simulink model "SecRwLtStHdrstUpwdDnwdTrgtPosSelc"  (R2018b)
settings: Solver=FixedStepDiscrete  StartTime=0.0  StopTime=10.0  FixedStep=0.01  RelTol=1e-3
undefined symbols (not defined in the file or in its folder): KeSMSw4SAcsMd21SecRwLtStHdrstUpwdDnwdPos_Val, KeSMSw4SAcsMd21SecRwLtStHdrstUpwdDnwdPosMax_Val, KeSMSw4SAcsMd21SecRwLtStHdrstUpwdDnwdPosMin_Val, KeSMSw4SAcsMd22SecRwLtStHdrstUpwdDnwdPos_Val, KeSMSw4SAcsMd22SecRwLtStHdrstUpwdDnwdPosMax_Val, KeSMSw4SAcsMd22SecRwLtStHdrstUpwdDnwdPosMin_Val, KeSMSw4SAcsMd25SecRwLtStHdrstUpwdDnwdPos_Val, KeSMSw4SAcsMd25SecRwLtStHdrstUpwdDnwdPosMax_Val, KeSMSw4SAcsMd25SecRwLtStHdrstUpwdDnwdPosMin_Val, KeSMSw4SAcsMd26SecRwLtStHdrstUpwdDnwdPos_Val, KeSMSw4SAcsMd26SecRwLtStHdrstUpwdDnwdPosMax_Val, KeSMSw4SAcsMd26SecRwLtStHdrstUpwdDnwdPosMin_Val, KeSMSw4sLyingMDSecRwLtStHdrstUpwdDnwdPos_160_Val, KeSMSw4sLyingMDSecRwLtStHdrstUpwdDnwdPos_165_Val, KeSMSw4sLyingMDSecRwLtStHdrstUpwdDnwdPos_170_Val, KeSMSw4sLyingMDSecRwLtStHdrstUpwdDnwdPos_175_Val, KeSMSw4sLyingMDSecRwLtStHdrstUpwdDnwdPos_180_Val, KeSMSw4sLyingMDSecRwLtStHdrstUpwdDnwdPos_Below160_Val, KeSMSw4sLyingMDSecRwLtStHdrstUpwdDnwdPos_Over180_Val, KeSMSw4sLyingMDSecRwLtStHdrstUpwdDnwdPosMax_160_Val, KeSMSw4sLyingMDSecRwLtStHdrstUpwdDnwdPosMax_165_Val, KeSMSw4sLyingMDSecRwLtStHdrstUpwdDnwdPosMax_170_Val, KeSMSw4sLyingMDSecRwLtStHdrstUpwdDnwdPosMax_175_Val, KeSMSw4sLyingMDSecRwLtStHdrstUpwdDnwdPosMax_180_Val, KeSMSw4sLyingMDSecRwLtStHdrstUpwdDnwdPosMax_Below160_Val, KeSMSw4sLyingMDSecRwLtStHdrstUpwdDnwdPosMax_Over180_Val, KeSMSw4sLyingMDSecRwLtStHdrstUpwdDnwdPosMin_160_Val, KeSMSw4sLyingMDSecRwLtStHdrstUpwdDnwdPosMin_165_Val, KeSMSw4sLyingMDSecRwLtStHdrstUpwdDnwdPosMin_170_Val, KeSMSw4sLyingMDSecRwLtStHdrstUpwdDnwdPosMin_175_Val, KeSMSw4sLyingMDSecRwLtStHdrstUpwdDnwdPosMin_180_Val, KeSMSw4sLyingMDSecRwLtStHdrstUpwdDnwdPosMin_Below160_Val, KeSMSw4sLyingMDSecRwLtStHdrstUpwdDnwdPosMin_Over180_Val, KeSMSw4sRecoveryMDSecRwLtStHdrstUpwdDnwdPos_160_Val, KeSMSw4sRecoveryMDSecRwLtStHdrstUpwdDnwdPos_165_Val, KeSMSw4sRecoveryMDSecRwLtStHdrstUpwdDnwdPos_170_Val, KeSMSw4sRecoveryMDSecRwLtStHdrstUpwdDnwdPos_175_Val, KeSMSw4sRecoveryMDSecRwLtStHdrstUpwdDnwdPos_180_Val, KeSMSw4sRecoveryMDSecRwLtStHdrstUpwdDnwdPos_Below160_Val, KeSMSw4sRecoveryMDSecRwLtStHdrstUpwdDnwdPos_Over180_Val, KeSMSw4sRecoveryMDSecRwLtStHdrstUpwdDnwdPosMax_160_Val, KeSMSw4sRecoveryMDSecRwLtStHdrstUpwdDnwdPosMax_165_Val, KeSMSw4sRecoveryMDSecRwLtStHdrstUpwdDnwdPosMax_170_Val, KeSMSw4sRecoveryMDSecRwLtStHdrstUpwdDnwdPosMax_175_Val, KeSMSw4sRecoveryMDSecRwLtStHdrstUpwdDnwdPosMax_180_Val, KeSMSw4sRecoveryMDSecRwLtStHdrstUpwdDnwdPosMax_Below160_Val, KeSMSw4sRecoveryMDSecRwLtStHdrstUpwdDnwdPosMax_Over180_Val, KeSMSw4sRecoveryMDSecRwLtStHdrstUpwdDnwdPosMin_160_Val, KeSMSw4sRecoveryMDSecRwLtStHdrstUpwdDnwdPosMin_165_Val, KeSMSw4sRecoveryMDSecRwLtStHdrstUpwdDnwdPosMin_170_Val, KeSMSw4sRecoveryMDSecRwLtStHdrstUpwdDnwdPosMin_175_Val, KeSMSw4sRecoveryMDSecRwLtStHdrstUpwdDnwdPosMin_180_Val, KeSMSw4sRecoveryMDSecRwLtStHdrstUpwdDnwdPosMin_Below160_Val, KeSMSw4sRecoveryMDSecRwLtStHdrstUpwdDnwdPosMin_Over180_Val, KeSMSw4sVIPMDSecRwLtStHdrstUpwdDnwdPos_160_Val, KeSMSw4sVIPMDSecRwLtStHdrstUpwdDnwdPos_165_Val, KeSMSw4sVIPMDSecRwLtStHdrstUpwdDnwdPos_170_Val, KeSMSw4sVIPMDSecRwLtStHdrstUpwdDnwdPos_175_Val, KeSMSw4sVIPMDSecRwLtStHdrstUpwdDnwdPos_180_Val, KeSMSw4sVIPMDSecRwLtStHdrstUpwdDnwdPos_Below160_Val ... (+15)
libraries: TrgtPosSelcLib x7
settings Model: ModifiedHistory=2023.8.1 V2.0.0 CR401790 增加模式21-26  Creator=sn2xws  LastModifiedBy=sn2xws
settings DataIOCC: SaveFormat=StructureWithTime
settings OptimizationCC: DefaultParameterBehavior=Inlined  EnhancedBackFolding=on  PassReuseOutputArgsAs=Individual arguments  ZeroExternalMemoryAtStartup=off  ZeroInternalMemoryAtStartup=off  OptimizeBlockOrder=speed  DifferentSizesBufferReuse=on  OptimizationCustomize=off
settings DebuggingCC: ParameterTunabilityLossMsg=error
settings ModelReferenceCC: ModelReferenceNumInstancesAllowed=Single
settings SFSimCC: MATLABDynamicMemAlloc=off
settings RTWCC: SystemTargetFile=autosar.tlc  GenCodeOnly=on  TemplateMakefile=ert_default_tmf  Description=AUTOSAR  GenerateReport=on  IncludeHyperlinkInReport=on  LaunchReport=on  GenerateTraceInfo=on  GenerateTraceReport=on  GenerateTraceReportSl=on  GenerateTraceReportSf=on  GenerateTraceReportEml=on  GenerateCodeMetricsReport=on
settings CodeAppCC: ForceParamTrailComments=on  IgnoreCustomStorageClasses=off  OperatorAnnotations=on  SimulinkDataObjDesc=on  SFDataObjDesc=on  InsertBlockDesc=on
settings STFCustomTargetCC: TargetLangStandard=C99 (ISO)  MultiwordLength=256  ParMdlRefBuildCompliant=on  CompOptLevelCompliant=on  IncludeMdlTerminateFcn=off  CombineOutputUpdateFcns=on  SuppressErrorStatus=on  ERTCustomFileBanners=on  SupportNonFinite=off  SupportComplex=off  SupportContinuousTime=off  SupportNonInlinedSFcns=off  RemoveResetFunc=on  MATLABClassNameForMDSCustomization=Simulink.SoftwareTarget.ERTCustomization  AutosarCompliant=on  UseToolchainInfoCompliant=on  LookupTableObjectStructAxisOrder=2,1,3,4,...  LUTObjectStructOrderEvenSpacing=Size,Table,Breakpoints  SystemTargetFile=autosar.tlc
settings ERTTargetCC: TargetLangStandard=C99 (ISO)  ConcurrentExecutionCompliant=off  IncludeMdlTerminateFcn=off  SuppressErrorStatus=on  SupportNonFinite=off  SupportComplex=off  ModelStepFunctionPrototypeControlCompliant=off  CPPClassGenCompliant=off  AutosarCompliant=on  LookupTableObjectStructAxisOrder=2,1,3,4,...  LUTObjectStructOrderEvenSpacing=Size,Table,Breakpoints  InlinedParameterPlacement=NonHierarchical  ERTCustomFileTemplate=example_file_process.tlc  ERTFilePackagingFormat=Compact

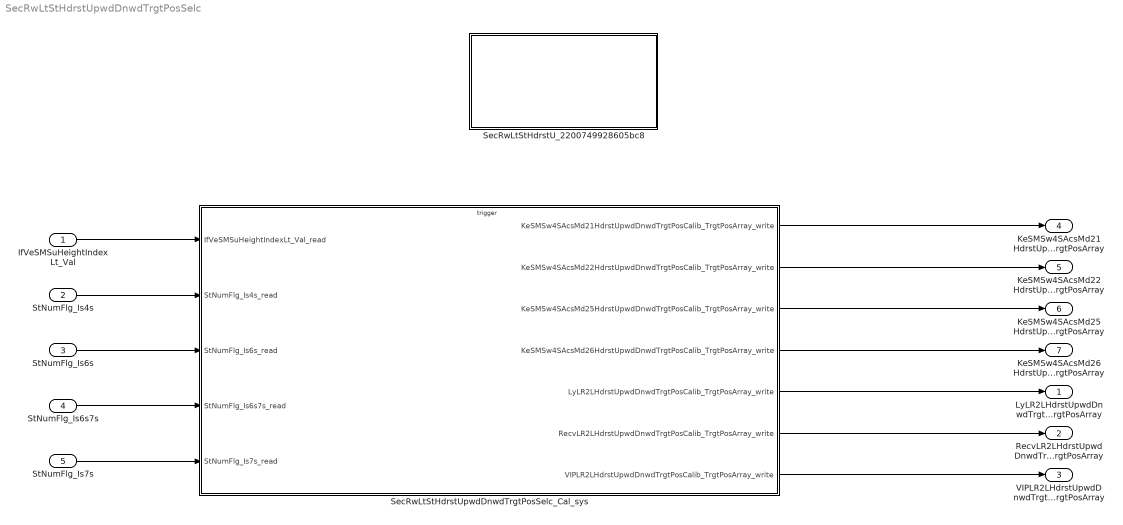
== system SecRwLtStHdrstUpwdDnwdTrgtPosSelc ==
  IfVeSMSuHeightIndexLt_Val : Inport  Description=|  OutDataTypeStr=uint8  PortDimensions=1
      | 0：under 160
      | 1：160
      | 2：165
      | 3：170
      | 4：175
      | 5：180
      | 6：over 180
  StNumFlg_Is4s : Inport  Port=2  OutDataTypeStr=boolean  PortDimensions=1
  StNumFlg_Is6s : Inport  Port=3  OutDataTypeStr=boolean  PortDimensions=1
  StNumFlg_Is6s7s : Inport  Port=4  OutDataTypeStr=boolean  PortDimensions=1
  StNumFlg_Is7s : Inport  Port=5  OutDataTypeStr=boolean  PortDimensions=1
  SecRwLtStHdrstU_2200749928605bc8 : Subsystem
  SecRwLtStHdrstUpwdDnwdTrgtPosSelc_Cal_sys : Subsystem
  LyLR2LHdrstUpwdDnwdTrgtPosCalib_TrgtPosArray : Outport  Description=|  OutDataTypeStr=uint16  PortDimensions=3
      | 0:Pos
      | 1:Max
      | 2:Min
  RecvLR2LHdrstUpwdDnwdTrgtPosCalib_TrgtPosArray : Outport  Description=|  Port=2  OutDataTypeStr=uint16  PortDimensions=3
      | 0:Pos
      | 1:Max
      | 2:Min
  VIPLR2LHdrstUpwdDnwdTrgtPosCalib_TrgtPosArray : Outport  Description=|  Port=3  OutDataTypeStr=uint16  PortDimensions=3
      | 0:Pos
      | 1:Max
      | 2:Min
  KeSMSw4SAcsMd21HdrstUpwdDnwdTrgtPosCalib_TrgtPosArray : Outport  Description=|  Port=4  OutDataTypeStr=uint16  PortDimensions=3
      | 0:Pos
      | 1:Max
      | 2:Min
  KeSMSw4SAcsMd22HdrstUpwdDnwdTrgtPosCalib_TrgtPosArray : Outport  Description=|  Port=5  OutDataTypeStr=uint16  PortDimensions=3
      | 0:Pos
      | 1:Max
      | 2:Min
  KeSMSw4SAcsMd25HdrstUpwdDnwdTrgtPosCalib_TrgtPosArray : Outport  Description=|  Port=6  OutDataTypeStr=uint16  PortDimensions=3
      | 0:Pos
      | 1:Max
      | 2:Min
  KeSMSw4SAcsMd26HdrstUpwdDnwdTrgtPosCalib_TrgtPosArray : Outport  Description=|  Port=7  OutDataTypeStr=uint16  PortDimensions=3
      | 0:Pos
      | 1:Max
      | 2:Min
  wires:
  IfVeSMSuHeightIndexLt_Val/1 -> SecRwLtStHdrstUpwdDnwdTrgtPosSelc_Cal_sys/1(IfVeSMSuHeightIndexLt_Val_read)
  StNumFlg_Is4s/1 -> SecRwLtStHdrstUpwdDnwdTrgtPosSelc_Cal_sys/2(StNumFlg_Is4s_read)
  StNumFlg_Is6s/1 -> SecRwLtStHdrstUpwdDnwdTrgtPosSelc_Cal_sys/3(StNumFlg_Is6s_read)
  StNumFlg_Is6s7s/1 -> SecRwLtStHdrstUpwdDnwdTrgtPosSelc_Cal_sys/4(StNumFlg_Is6s7s_read)
  StNumFlg_Is7s/1 -> SecRwLtStHdrstUpwdDnwdTrgtPosSelc_Cal_sys/5(StNumFlg_Is7s_read)
  SecRwLtStHdrstUpwdDnwdTrgtPosSelc_Cal_sys/5(LyLR2LHdrstUpwdDnwdTrgtPosCalib_TrgtPosArray_write) -> LyLR2LHdrstUpwdDnwdTrgtPosCalib_TrgtPosArray/1
  SecRwLtStHdrstUpwdDnwdTrgtPosSelc_Cal_sys/6(RecvLR2LHdrstUpwdDnwdTrgtPosCalib_TrgtPosArray_write) -> RecvLR2LHdrstUpwdDnwdTrgtPosCalib_TrgtPosArray/1
  SecRwLtStHdrstUpwdDnwdTrgtPosSelc_Cal_sys/7(VIPLR2LHdrstUpwdDnwdTrgtPosCalib_TrgtPosArray_write) -> VIPLR2LHdrstUpwdDnwdTrgtPosCalib_TrgtPosArray/1
  SecRwLtStHdrstUpwdDnwdTrgtPosSelc_Cal_sys/1(KeSMSw4SAcsMd21HdrstUpwdDnwdTrgtPosCalib_TrgtPosArray_write) -> KeSMSw4SAcsMd21HdrstUpwdDnwdTrgtPosCalib_TrgtPosArray/1
  SecRwLtStHdrstUpwdDnwdTrgtPosSelc_Cal_sys/2(KeSMSw4SAcsMd22HdrstUpwdDnwdTrgtPosCalib_TrgtPosArray_write) -> KeSMSw4SAcsMd22HdrstUpwdDnwdTrgtPosCalib_TrgtPosArray/1
  SecRwLtStHdrstUpwdDnwdTrgtPosSelc_Cal_sys/3(KeSMSw4SAcsMd25HdrstUpwdDnwdTrgtPosCalib_TrgtPosArray_write) -> KeSMSw4SAcsMd25HdrstUpwdDnwdTrgtPosCalib_TrgtPosArray/1
  SecRwLtStHdrstUpwdDnwdTrgtPosSelc_Cal_sys/4(KeSMSw4SAcsMd26HdrstUpwdDnwdTrgtPosCalib_TrgtPosArray_write) -> KeSMSw4SAcsMd26HdrstUpwdDnwdTrgtPosCalib_TrgtPosArray/1

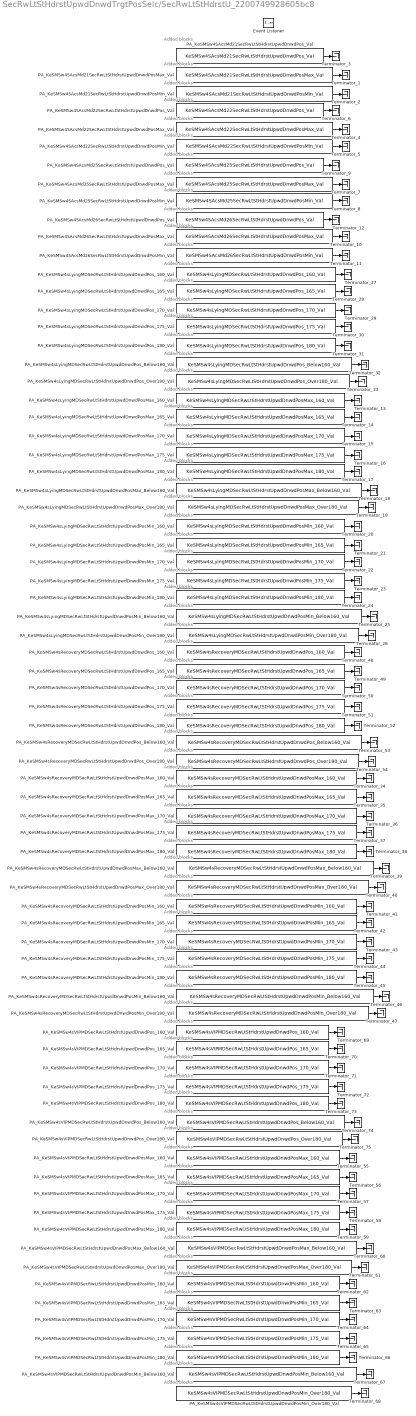
== system SecRwLtStHdrstUpwdDnwdTrgtPosSelc/SecRwLtStHdrstU_2200749928605bc8 ==
  note: Added blocks
  note: Added blocks
  note: Added blocks
  note: Added blocks
  note: Added blocks
  note: Added blocks
  note: Added blocks
  note: Added blocks
  note: Added blocks
  note: Added blocks
  note: Added blocks
  note: Added blocks
  note: Added blocks
  note: Added blocks
  note: Added blocks
  note: Added blocks
  note: Added blocks
  note: Added blocks
  note: Added blocks
  note: Added blocks
  note: Added blocks
  note: Added blocks
  note: Added blocks
  note: Added blocks
  note: Added blocks
  note: Added blocks
  note: Added blocks
  note: Added blocks
  note: Added blocks
  note: Added blocks
  note: Added blocks
  note: Added blocks
  note: Added blocks
  note: Added blocks
  note: Added blocks
  note: Added blocks
  note: Added blocks
  note: Added blocks
  note: Added blocks
  note: Added blocks
  note: Added blocks
  note: Added blocks
  note: Added blocks
  note: Added blocks
  note: Added blocks
  note: Added blocks
  note: Added blocks
  note: Added blocks
  note: Added blocks
  note: Added blocks
  note: Added blocks
  note: Added blocks
  note: Added blocks
  note: Added blocks
  note: Added blocks
  note: Added blocks
  note: Added blocks
  note: Added blocks
  note: Added blocks
  note: Added blocks
  note: Added blocks
  note: Added blocks
  note: Added blocks
  note: Added blocks
  note: Added blocks
  note: Added blocks
  note: Added blocks
  note: Added blocks
  note: Added blocks
  note: Added blocks
  note: Added blocks
  note: Added blocks
  note: Added blocks
  note: Added blocks
  note: Added blocks
  Event Listener : EventListener  EventName=reset
  PA_KeSMSw4SAcsMd21SecRwLtStHdrstUpwdDnwdPosMax_Val : Constant  Value=KeSMSw4SAcsMd21SecRwLtStHdrstUpwdDnwdPosMax_Val
  PA_KeSMSw4SAcsMd21SecRwLtStHdrstUpwdDnwdPosMin_Val : Constant  Value=KeSMSw4SAcsMd21SecRwLtStHdrstUpwdDnwdPosMin_Val
  PA_KeSMSw4SAcsMd21SecRwLtStHdrstUpwdDnwdPos_Val : Constant  Value=KeSMSw4SAcsMd21SecRwLtStHdrstUpwdDnwdPos_Val
  PA_KeSMSw4SAcsMd22SecRwLtStHdrstUpwdDnwdPosMax_Val : Constant  Value=KeSMSw4SAcsMd22SecRwLtStHdrstUpwdDnwdPosMax_Val
  PA_KeSMSw4SAcsMd22SecRwLtStHdrstUpwdDnwdPosMin_Val : Constant  Value=KeSMSw4SAcsMd22SecRwLtStHdrstUpwdDnwdPosMin_Val
  PA_KeSMSw4SAcsMd22SecRwLtStHdrstUpwdDnwdPos_Val : Constant  Value=KeSMSw4SAcsMd22SecRwLtStHdrstUpwdDnwdPos_Val
  PA_KeSMSw4SAcsMd25SecRwLtStHdrstUpwdDnwdPosMax_Val : Constant  Value=KeSMSw4SAcsMd25SecRwLtStHdrstUpwdDnwdPosMax_Val
  PA_KeSMSw4SAcsMd25SecRwLtStHdrstUpwdDnwdPosMin_Val : Constant  Value=KeSMSw4SAcsMd25SecRwLtStHdrstUpwdDnwdPosMin_Val
  PA_KeSMSw4SAcsMd25SecRwLtStHdrstUpwdDnwdPos_Val : Constant  Value=KeSMSw4SAcsMd25SecRwLtStHdrstUpwdDnwdPos_Val
  PA_KeSMSw4SAcsMd26SecRwLtStHdrstUpwdDnwdPosMax_Val : Constant  Value=KeSMSw4SAcsMd26SecRwLtStHdrstUpwdDnwdPosMax_Val
  PA_KeSMSw4SAcsMd26SecRwLtStHdrstUpwdDnwdPosMin_Val : Constant  Value=KeSMSw4SAcsMd26SecRwLtStHdrstUpwdDnwdPosMin_Val
  PA_KeSMSw4SAcsMd26SecRwLtStHdrstUpwdDnwdPos_Val : Constant  Value=KeSMSw4SAcsMd26SecRwLtStHdrstUpwdDnwdPos_Val
  PA_KeSMSw4sLyingMDSecRwLtStHdrstUpwdDnwdPosMax_160_Val : Constant  Value=KeSMSw4sLyingMDSecRwLtStHdrstUpwdDnwdPosMax_160_Val
  PA_KeSMSw4sLyingMDSecRwLtStHdrstUpwdDnwdPosMax_165_Val : Constant  Value=KeSMSw4sLyingMDSecRwLtStHdrstUpwdDnwdPosMax_165_Val
  PA_KeSMSw4sLyingMDSecRwLtStHdrstUpwdDnwdPosMax_170_Val : Constant  Value=KeSMSw4sLyingMDSecRwLtStHdrstUpwdDnwdPosMax_170_Val
  PA_KeSMSw4sLyingMDSecRwLtStHdrstUpwdDnwdPosMax_175_Val : Constant  Value=KeSMSw4sLyingMDSecRwLtStHdrstUpwdDnwdPosMax_175_Val
  PA_KeSMSw4sLyingMDSecRwLtStHdrstUpwdDnwdPosMax_180_Val : Constant  Value=KeSMSw4sLyingMDSecRwLtStHdrstUpwdDnwdPosMax_180_Val
  PA_KeSMSw4sLyingMDSecRwLtStHdrstUpwdDnwdPosMax_Below160_Val : Constant  Value=KeSMSw4sLyingMDSecRwLtStHdrstUpwdDnwdPosMax_Below160_Val
  PA_KeSMSw4sLyingMDSecRwLtStHdrstUpwdDnwdPosMax_Over180_Val : Constant  Value=KeSMSw4sLyingMDSecRwLtStHdrstUpwdDnwdPosMax_Over180_Val
  PA_KeSMSw4sLyingMDSecRwLtStHdrstUpwdDnwdPosMin_160_Val : Constant  Value=KeSMSw4sLyingMDSecRwLtStHdrstUpwdDnwdPosMin_160_Val
  PA_KeSMSw4sLyingMDSecRwLtStHdrstUpwdDnwdPosMin_165_Val : Constant  Value=KeSMSw4sLyingMDSecRwLtStHdrstUpwdDnwdPosMin_165_Val
  PA_KeSMSw4sLyingMDSecRwLtStHdrstUpwdDnwdPosMin_170_Val : Constant  Value=KeSMSw4sLyingMDSecRwLtStHdrstUpwdDnwdPosMin_170_Val
  PA_KeSMSw4sLyingMDSecRwLtStHdrstUpwdDnwdPosMin_175_Val : Constant  Value=KeSMSw4sLyingMDSecRwLtStHdrstUpwdDnwdPosMin_175_Val
  PA_KeSMSw4sLyingMDSecRwLtStHdrstUpwdDnwdPosMin_180_Val : Constant  Value=KeSMSw4sLyingMDSecRwLtStHdrstUpwdDnwdPosMin_180_Val
  PA_KeSMSw4sLyingMDSecRwLtStHdrstUpwdDnwdPosMin_Below160_Val : Constant  Value=KeSMSw4sLyingMDSecRwLtStHdrstUpwdDnwdPosMin_Below160_Val
  PA_KeSMSw4sLyingMDSecRwLtStHdrstUpwdDnwdPosMin_Over180_Val : Constant  Value=KeSMSw4sLyingMDSecRwLtStHdrstUpwdDnwdPosMin_Over180_Val
  PA_KeSMSw4sLyingMDSecRwLtStHdrstUpwdDnwdPos_160_Val : Constant  Value=KeSMSw4sLyingMDSecRwLtStHdrstUpwdDnwdPos_160_Val
  PA_KeSMSw4sLyingMDSecRwLtStHdrstUpwdDnwdPos_165_Val : Constant  Value=KeSMSw4sLyingMDSecRwLtStHdrstUpwdDnwdPos_165_Val
  PA_KeSMSw4sLyingMDSecRwLtStHdrstUpwdDnwdPos_170_Val : Constant  Value=KeSMSw4sLyingMDSecRwLtStHdrstUpwdDnwdPos_170_Val
  PA_KeSMSw4sLyingMDSecRwLtStHdrstUpwdDnwdPos_175_Val : Constant  Value=KeSMSw4sLyingMDSecRwLtStHdrstUpwdDnwdPos_175_Val
  PA_KeSMSw4sLyingMDSecRwLtStHdrstUpwdDnwdPos_180_Val : Constant  Value=KeSMSw4sLyingMDSecRwLtStHdrstUpwdDnwdPos_180_Val
  PA_KeSMSw4sLyingMDSecRwLtStHdrstUpwdDnwdPos_Below160_Val : Constant  Value=KeSMSw4sLyingMDSecRwLtStHdrstUpwdDnwdPos_Below160_Val
  PA_KeSMSw4sLyingMDSecRwLtStHdrstUpwdDnwdPos_Over180_Val : Constant  Value=KeSMSw4sLyingMDSecRwLtStHdrstUpwdDnwdPos_Over180_Val
  PA_KeSMSw4sRecoveryMDSecRwLtStHdrstUpwdDnwdPosMax_160_Val : Constant  Value=KeSMSw4sRecoveryMDSecRwLtStHdrstUpwdDnwdPosMax_160_Val
  PA_KeSMSw4sRecoveryMDSecRwLtStHdrstUpwdDnwdPosMax_165_Val : Constant  Value=KeSMSw4sRecoveryMDSecRwLtStHdrstUpwdDnwdPosMax_165_Val
  PA_KeSMSw4sRecoveryMDSecRwLtStHdrstUpwdDnwdPosMax_170_Val : Constant  Value=KeSMSw4sRecoveryMDSecRwLtStHdrstUpwdDnwdPosMax_170_Val
  PA_KeSMSw4sRecoveryMDSecRwLtStHdrstUpwdDnwdPosMax_175_Val : Constant  Value=KeSMSw4sRecoveryMDSecRwLtStHdrstUpwdDnwdPosMax_175_Val
  PA_KeSMSw4sRecoveryMDSecRwLtStHdrstUpwdDnwdPosMax_180_Val : Constant  Value=KeSMSw4sRecoveryMDSecRwLtStHdrstUpwdDnwdPosMax_180_Val
  PA_KeSMSw4sRecoveryMDSecRwLtStHdrstUpwdDnwdPosMax_Below160_Val : Constant  Value=KeSMSw4sRecoveryMDSecRwLtStHdrstUpwdDnwdPosMax_Below160_Val
  PA_KeSMSw4sRecoveryMDSecRwLtStHdrstUpwdDnwdPosMax_Over180_Val : Constant  Value=KeSMSw4sRecoveryMDSecRwLtStHdrstUpwdDnwdPosMax_Over180_Val
  PA_KeSMSw4sRecoveryMDSecRwLtStHdrstUpwdDnwdPosMin_160_Val : Constant  Value=KeSMSw4sRecoveryMDSecRwLtStHdrstUpwdDnwdPosMin_160_Val
  PA_KeSMSw4sRecoveryMDSecRwLtStHdrstUpwdDnwdPosMin_165_Val : Constant  Value=KeSMSw4sRecoveryMDSecRwLtStHdrstUpwdDnwdPosMin_165_Val
  PA_KeSMSw4sRecoveryMDSecRwLtStHdrstUpwdDnwdPosMin_170_Val : Constant  Value=KeSMSw4sRecoveryMDSecRwLtStHdrstUpwdDnwdPosMin_170_Val
  PA_KeSMSw4sRecoveryMDSecRwLtStHdrstUpwdDnwdPosMin_175_Val : Constant  Value=KeSMSw4sRecoveryMDSecRwLtStHdrstUpwdDnwdPosMin_175_Val
  PA_KeSMSw4sRecoveryMDSecRwLtStHdrstUpwdDnwdPosMin_180_Val : Constant  Value=KeSMSw4sRecoveryMDSecRwLtStHdrstUpwdDnwdPosMin_180_Val
  PA_KeSMSw4sRecoveryMDSecRwLtStHdrstUpwdDnwdPosMin_Below160_Val : Constant  Value=KeSMSw4sRecoveryMDSecRwLtStHdrstUpwdDnwdPosMin_Below160_Val
  PA_KeSMSw4sRecoveryMDSecRwLtStHdrstUpwdDnwdPosMin_Over180_Val : Constant  Value=KeSMSw4sRecoveryMDSecRwLtStHdrstUpwdDnwdPosMin_Over180_Val
  PA_KeSMSw4sRecoveryMDSecRwLtStHdrstUpwdDnwdPos_160_Val : Constant  Value=KeSMSw4sRecoveryMDSecRwLtStHdrstUpwdDnwdPos_160_Val
  PA_KeSMSw4sRecoveryMDSecRwLtStHdrstUpwdDnwdPos_165_Val : Constant  Value=KeSMSw4sRecoveryMDSecRwLtStHdrstUpwdDnwdPos_165_Val
  PA_KeSMSw4sRecoveryMDSecRwLtStHdrstUpwdDnwdPos_170_Val : Constant  Value=KeSMSw4sRecoveryMDSecRwLtStHdrstUpwdDnwdPos_170_Val
  PA_KeSMSw4sRecoveryMDSecRwLtStHdrstUpwdDnwdPos_175_Val : Constant  Value=KeSMSw4sRecoveryMDSecRwLtStHdrstUpwdDnwdPos_175_Val
  PA_KeSMSw4sRecoveryMDSecRwLtStHdrstUpwdDnwdPos_180_Val : Constant  Value=KeSMSw4sRecoveryMDSecRwLtStHdrstUpwdDnwdPos_180_Val
  PA_KeSMSw4sRecoveryMDSecRwLtStHdrstUpwdDnwdPos_Below160_Val : Constant  Value=KeSMSw4sRecoveryMDSecRwLtStHdrstUpwdDnwdPos_Below160_Val
  PA_KeSMSw4sRecoveryMDSecRwLtStHdrstUpwdDnwdPos_Over180_Val : Constant  Value=KeSMSw4sRecoveryMDSecRwLtStHdrstUpwdDnwdPos_Over180_Val
  PA_KeSMSw4sVIPMDSecRwLtStHdrstUpwdDnwdPosMax_160_Val : Constant  Value=KeSMSw4sVIPMDSecRwLtStHdrstUpwdDnwdPosMax_160_Val
  PA_KeSMSw4sVIPMDSecRwLtStHdrstUpwdDnwdPosMax_165_Val : Constant  Value=KeSMSw4sVIPMDSecRwLtStHdrstUpwdDnwdPosMax_165_Val
  PA_KeSMSw4sVIPMDSecRwLtStHdrstUpwdDnwdPosMax_170_Val : Constant  Value=KeSMSw4sVIPMDSecRwLtStHdrstUpwdDnwdPosMax_170_Val
  PA_KeSMSw4sVIPMDSecRwLtStHdrstUpwdDnwdPosMax_175_Val : Constant  Value=KeSMSw4sVIPMDSecRwLtStHdrstUpwdDnwdPosMax_175_Val
  PA_KeSMSw4sVIPMDSecRwLtStHdrstUpwdDnwdPosMax_180_Val : Constant  Value=KeSMSw4sVIPMDSecRwLtStHdrstUpwdDnwdPosMax_180_Val
  PA_KeSMSw4sVIPMDSecRwLtStHdrstUpwdDnwdPosMax_Below160_Val : Constant  Value=KeSMSw4sVIPMDSecRwLtStHdrstUpwdDnwdPosMax_Below160_Val
  PA_KeSMSw4sVIPMDSecRwLtStHdrstUpwdDnwdPosMax_Over180_Val : Constant  Value=KeSMSw4sVIPMDSecRwLtStHdrstUpwdDnwdPosMax_Over180_Val
  PA_KeSMSw4sVIPMDSecRwLtStHdrstUpwdDnwdPosMin_160_Val : Constant  Value=KeSMSw4sVIPMDSecRwLtStHdrstUpwdDnwdPosMin_160_Val
  PA_KeSMSw4sVIPMDSecRwLtStHdrstUpwdDnwdPosMin_165_Val : Constant  Value=KeSMSw4sVIPMDSecRwLtStHdrstUpwdDnwdPosMin_165_Val
  PA_KeSMSw4sVIPMDSecRwLtStHdrstUpwdDnwdPosMin_170_Val : Constant  Value=KeSMSw4sVIPMDSecRwLtStHdrstUpwdDnwdPosMin_170_Val
  PA_KeSMSw4sVIPMDSecRwLtStHdrstUpwdDnwdPosMin_175_Val : Constant  Value=KeSMSw4sVIPMDSecRwLtStHdrstUpwdDnwdPosMin_175_Val
  PA_KeSMSw4sVIPMDSecRwLtStHdrstUpwdDnwdPosMin_180_Val : Constant  Value=KeSMSw4sVIPMDSecRwLtStHdrstUpwdDnwdPosMin_180_Val
  PA_KeSMSw4sVIPMDSecRwLtStHdrstUpwdDnwdPosMin_Below160_Val : Constant  Value=KeSMSw4sVIPMDSecRwLtStHdrstUpwdDnwdPosMin_Below160_Val
  PA_KeSMSw4sVIPMDSecRwLtStHdrstUpwdDnwdPosMin_Over180_Val : Constant  Value=KeSMSw4sVIPMDSecRwLtStHdrstUpwdDnwdPosMin_Over180_Val
  PA_KeSMSw4sVIPMDSecRwLtStHdrstUpwdDnwdPos_160_Val : Constant  Value=KeSMSw4sVIPMDSecRwLtStHdrstUpwdDnwdPos_160_Val
  PA_KeSMSw4sVIPMDSecRwLtStHdrstUpwdDnwdPos_165_Val : Constant  Value=KeSMSw4sVIPMDSecRwLtStHdrstUpwdDnwdPos_165_Val
  PA_KeSMSw4sVIPMDSecRwLtStHdrstUpwdDnwdPos_170_Val : Constant  Value=KeSMSw4sVIPMDSecRwLtStHdrstUpwdDnwdPos_170_Val
  PA_KeSMSw4sVIPMDSecRwLtStHdrstUpwdDnwdPos_175_Val : Constant  Value=KeSMSw4sVIPMDSecRwLtStHdrstUpwdDnwdPos_175_Val
  PA_KeSMSw4sVIPMDSecRwLtStHdrstUpwdDnwdPos_180_Val : Constant  Value=KeSMSw4sVIPMDSecRwLtStHdrstUpwdDnwdPos_180_Val
  PA_KeSMSw4sVIPMDSecRwLtStHdrstUpwdDnwdPos_Below160_Val : Constant  Value=KeSMSw4sVIPMDSecRwLtStHdrstUpwdDnwdPos_Below160_Val
  PA_KeSMSw4sVIPMDSecRwLtStHdrstUpwdDnwdPos_Over180_Val : Constant  Value=KeSMSw4sVIPMDSecRwLtStHdrstUpwdDnwdPos_Over180_Val
  Terminator_{1..75} (75 alike) : Terminator
  wires:
  PA_KeSMSw4SAcsMd21SecRwLtStHdrstUpwdDnwdPosMax_Val/1 -> Terminator_1/1
  PA_KeSMSw4SAcsMd21SecRwLtStHdrstUpwdDnwdPosMin_Val/1 -> Terminator_2/1
  PA_KeSMSw4SAcsMd21SecRwLtStHdrstUpwdDnwdPos_Val/1 -> Terminator_3/1
  PA_KeSMSw4SAcsMd22SecRwLtStHdrstUpwdDnwdPosMax_Val/1 -> Terminator_4/1
  PA_KeSMSw4SAcsMd22SecRwLtStHdrstUpwdDnwdPosMin_Val/1 -> Terminator_5/1
  PA_KeSMSw4SAcsMd22SecRwLtStHdrstUpwdDnwdPos_Val/1 -> Terminator_6/1
  PA_KeSMSw4SAcsMd25SecRwLtStHdrstUpwdDnwdPosMax_Val/1 -> Terminator_7/1
  PA_KeSMSw4SAcsMd25SecRwLtStHdrstUpwdDnwdPosMin_Val/1 -> Terminator_8/1
  PA_KeSMSw4SAcsMd25SecRwLtStHdrstUpwdDnwdPos_Val/1 -> Terminator_9/1
  PA_KeSMSw4SAcsMd26SecRwLtStHdrstUpwdDnwdPosMax_Val/1 -> Terminator_10/1
  PA_KeSMSw4SAcsMd26SecRwLtStHdrstUpwdDnwdPosMin_Val/1 -> Terminator_11/1
  PA_KeSMSw4SAcsMd26SecRwLtStHdrstUpwdDnwdPos_Val/1 -> Terminator_12/1
  PA_KeSMSw4sLyingMDSecRwLtStHdrstUpwdDnwdPosMax_160_Val/1 -> Terminator_13/1
  PA_KeSMSw4sLyingMDSecRwLtStHdrstUpwdDnwdPosMax_165_Val/1 -> Terminator_14/1
  PA_KeSMSw4sLyingMDSecRwLtStHdrstUpwdDnwdPosMax_170_Val/1 -> Terminator_15/1
  PA_KeSMSw4sLyingMDSecRwLtStHdrstUpwdDnwdPosMax_175_Val/1 -> Terminator_16/1
  PA_KeSMSw4sLyingMDSecRwLtStHdrstUpwdDnwdPosMax_180_Val/1 -> Terminator_17/1
  PA_KeSMSw4sLyingMDSecRwLtStHdrstUpwdDnwdPosMax_Below160_Val/1 -> Terminator_18/1
  PA_KeSMSw4sLyingMDSecRwLtStHdrstUpwdDnwdPosMax_Over180_Val/1 -> Terminator_19/1
  PA_KeSMSw4sLyingMDSecRwLtStHdrstUpwdDnwdPosMin_160_Val/1 -> Terminator_20/1
  PA_KeSMSw4sLyingMDSecRwLtStHdrstUpwdDnwdPosMin_165_Val/1 -> Terminator_21/1
  PA_KeSMSw4sLyingMDSecRwLtStHdrstUpwdDnwdPosMin_170_Val/1 -> Terminator_22/1
  PA_KeSMSw4sLyingMDSecRwLtStHdrstUpwdDnwdPosMin_175_Val/1 -> Terminator_23/1
  PA_KeSMSw4sLyingMDSecRwLtStHdrstUpwdDnwdPosMin_180_Val/1 -> Terminator_24/1
  PA_KeSMSw4sLyingMDSecRwLtStHdrstUpwdDnwdPosMin_Below160_Val/1 -> Terminator_25/1
  PA_KeSMSw4sLyingMDSecRwLtStHdrstUpwdDnwdPosMin_Over180_Val/1 -> Terminator_26/1
  PA_KeSMSw4sLyingMDSecRwLtStHdrstUpwdDnwdPos_160_Val/1 -> Terminator_27/1
  PA_KeSMSw4sLyingMDSecRwLtStHdrstUpwdDnwdPos_165_Val/1 -> Terminator_28/1
  PA_KeSMSw4sLyingMDSecRwLtStHdrstUpwdDnwdPos_170_Val/1 -> Terminator_29/1
  PA_KeSMSw4sLyingMDSecRwLtStHdrstUpwdDnwdPos_175_Val/1 -> Terminator_30/1
  PA_KeSMSw4sLyingMDSecRwLtStHdrstUpwdDnwdPos_180_Val/1 -> Terminator_31/1
  PA_KeSMSw4sLyingMDSecRwLtStHdrstUpwdDnwdPos_Below160_Val/1 -> Terminator_32/1
  PA_KeSMSw4sLyingMDSecRwLtStHdrstUpwdDnwdPos_Over180_Val/1 -> Terminator_33/1
  PA_KeSMSw4sRecoveryMDSecRwLtStHdrstUpwdDnwdPosMax_160_Val/1 -> Terminator_34/1
  PA_KeSMSw4sRecoveryMDSecRwLtStHdrstUpwdDnwdPosMax_165_Val/1 -> Terminator_35/1
  PA_KeSMSw4sRecoveryMDSecRwLtStHdrstUpwdDnwdPosMax_170_Val/1 -> Terminator_36/1
  PA_KeSMSw4sRecoveryMDSecRwLtStHdrstUpwdDnwdPosMax_175_Val/1 -> Terminator_37/1
  PA_KeSMSw4sRecoveryMDSecRwLtStHdrstUpwdDnwdPosMax_180_Val/1 -> Terminator_38/1
  PA_KeSMSw4sRecoveryMDSecRwLtStHdrstUpwdDnwdPosMax_Below160_Val/1 -> Terminator_39/1
  PA_KeSMSw4sRecoveryMDSecRwLtStHdrstUpwdDnwdPosMax_Over180_Val/1 -> Terminator_40/1
  PA_KeSMSw4sRecoveryMDSecRwLtStHdrstUpwdDnwdPosMin_160_Val/1 -> Terminator_41/1
  PA_KeSMSw4sRecoveryMDSecRwLtStHdrstUpwdDnwdPosMin_165_Val/1 -> Terminator_42/1
  PA_KeSMSw4sRecoveryMDSecRwLtStHdrstUpwdDnwdPosMin_170_Val/1 -> Terminator_43/1
  PA_KeSMSw4sRecoveryMDSecRwLtStHdrstUpwdDnwdPosMin_175_Val/1 -> Terminator_44/1
  PA_KeSMSw4sRecoveryMDSecRwLtStHdrstUpwdDnwdPosMin_180_Val/1 -> Terminator_45/1
  PA_KeSMSw4sRecoveryMDSecRwLtStHdrstUpwdDnwdPosMin_Below160_Val/1 -> Terminator_46/1
  PA_KeSMSw4sRecoveryMDSecRwLtStHdrstUpwdDnwdPosMin_Over180_Val/1 -> Terminator_47/1
  PA_KeSMSw4sRecoveryMDSecRwLtStHdrstUpwdDnwdPos_160_Val/1 -> Terminator_48/1
  PA_KeSMSw4sRecoveryMDSecRwLtStHdrstUpwdDnwdPos_165_Val/1 -> Terminator_49/1
  PA_KeSMSw4sRecoveryMDSecRwLtStHdrstUpwdDnwdPos_170_Val/1 -> Terminator_50/1
  PA_KeSMSw4sRecoveryMDSecRwLtStHdrstUpwdDnwdPos_175_Val/1 -> Terminator_51/1
  PA_KeSMSw4sRecoveryMDSecRwLtStHdrstUpwdDnwdPos_180_Val/1 -> Terminator_52/1
  PA_KeSMSw4sRecoveryMDSecRwLtStHdrstUpwdDnwdPos_Below160_Val/1 -> Terminator_53/1
  PA_KeSMSw4sRecoveryMDSecRwLtStHdrstUpwdDnwdPos_Over180_Val/1 -> Terminator_54/1
  PA_KeSMSw4sVIPMDSecRwLtStHdrstUpwdDnwdPosMax_160_Val/1 -> Terminator_55/1
  PA_KeSMSw4sVIPMDSecRwLtStHdrstUpwdDnwdPosMax_165_Val/1 -> Terminator_56/1
  PA_KeSMSw4sVIPMDSecRwLtStHdrstUpwdDnwdPosMax_170_Val/1 -> Terminator_57/1
  PA_KeSMSw4sVIPMDSecRwLtStHdrstUpwdDnwdPosMax_175_Val/1 -> Terminator_58/1
  PA_KeSMSw4sVIPMDSecRwLtStHdrstUpwdDnwdPosMax_180_Val/1 -> Terminator_59/1
  PA_KeSMSw4sVIPMDSecRwLtStHdrstUpwdDnwdPosMax_Below160_Val/1 -> Terminator_60/1
  PA_KeSMSw4sVIPMDSecRwLtStHdrstUpwdDnwdPosMax_Over180_Val/1 -> Terminator_61/1
  PA_KeSMSw4sVIPMDSecRwLtStHdrstUpwdDnwdPosMin_160_Val/1 -> Terminator_62/1
  PA_KeSMSw4sVIPMDSecRwLtStHdrstUpwdDnwdPosMin_165_Val/1 -> Terminator_63/1
  PA_KeSMSw4sVIPMDSecRwLtStHdrstUpwdDnwdPosMin_170_Val/1 -> Terminator_64/1
  PA_KeSMSw4sVIPMDSecRwLtStHdrstUpwdDnwdPosMin_175_Val/1 -> Terminator_65/1
  PA_KeSMSw4sVIPMDSecRwLtStHdrstUpwdDnwdPosMin_180_Val/1 -> Terminator_66/1
  PA_KeSMSw4sVIPMDSecRwLtStHdrstUpwdDnwdPosMin_Below160_Val/1 -> Terminator_67/1
  PA_KeSMSw4sVIPMDSecRwLtStHdrstUpwdDnwdPosMin_Over180_Val/1 -> Terminator_68/1
  PA_KeSMSw4sVIPMDSecRwLtStHdrstUpwdDnwdPos_160_Val/1 -> Terminator_69/1
  PA_KeSMSw4sVIPMDSecRwLtStHdrstUpwdDnwdPos_165_Val/1 -> Terminator_70/1
  PA_KeSMSw4sVIPMDSecRwLtStHdrstUpwdDnwdPos_170_Val/1 -> Terminator_71/1
  PA_KeSMSw4sVIPMDSecRwLtStHdrstUpwdDnwdPos_175_Val/1 -> Terminator_72/1
  PA_KeSMSw4sVIPMDSecRwLtStHdrstUpwdDnwdPos_180_Val/1 -> Terminator_73/1
  PA_KeSMSw4sVIPMDSecRwLtStHdrstUpwdDnwdPos_Below160_Val/1 -> Terminator_74/1
  PA_KeSMSw4sVIPMDSecRwLtStHdrstUpwdDnwdPos_Over180_Val/1 -> Terminator_75/1

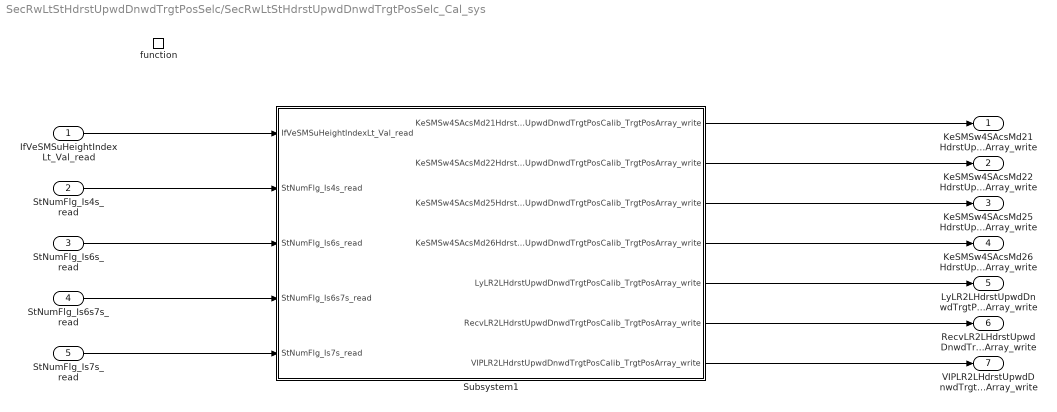
== system SecRwLtStHdrstUpwdDnwdTrgtPosSelc/SecRwLtStHdrstUpwdDnwdTrgtPosSelc_Cal_sys ==
  IfVeSMSuHeightIndexLt_Val_read : Inport
  StNumFlg_Is4s_read : Inport  Port=2
  StNumFlg_Is6s_read : Inport  Port=3
  StNumFlg_Is6s7s_read : Inport  Port=4
  StNumFlg_Is7s_read : Inport  Port=5
  function : TriggerPort  TriggerType=function-call  IsSimulinkFunction=on  FunctionName=SecRwLtStHdrstUpwdDnwdTrgtPosSelc_Cal  VariantControl=(inherit)
  Subsystem1 : Subsystem
  KeSMSw4SAcsMd21HdrstUpwdDnwdTrgtPosCalib_TrgtPosArray_write : Outport
      settings: EnsureOutportIsVirtual=on
  KeSMSw4SAcsMd22HdrstUpwdDnwdTrgtPosCalib_TrgtPosArray_write : Outport  Port=2
      settings: EnsureOutportIsVirtual=on
  KeSMSw4SAcsMd25HdrstUpwdDnwdTrgtPosCalib_TrgtPosArray_write : Outport  Port=3
      settings: EnsureOutportIsVirtual=on
  KeSMSw4SAcsMd26HdrstUpwdDnwdTrgtPosCalib_TrgtPosArray_write : Outport  Port=4
      settings: EnsureOutportIsVirtual=on
  LyLR2LHdrstUpwdDnwdTrgtPosCalib_TrgtPosArray_write : Outport  Port=5
      settings: EnsureOutportIsVirtual=on
  RecvLR2LHdrstUpwdDnwdTrgtPosCalib_TrgtPosArray_write : Outport  Port=6
      settings: EnsureOutportIsVirtual=on
  VIPLR2LHdrstUpwdDnwdTrgtPosCalib_TrgtPosArray_write : Outport  Port=7
      settings: EnsureOutportIsVirtual=on
  wires:
  Subsystem1/1(KeSMSw4SAcsMd21HdrstUpwdDnwdTrgtPosCalib_TrgtPosArray_write) -> KeSMSw4SAcsMd21HdrstUpwdDnwdTrgtPosCalib_TrgtPosArray_write/1
  Subsystem1/2(KeSMSw4SAcsMd22HdrstUpwdDnwdTrgtPosCalib_TrgtPosArray_write) -> KeSMSw4SAcsMd22HdrstUpwdDnwdTrgtPosCalib_TrgtPosArray_write/1
  Subsystem1/3(KeSMSw4SAcsMd25HdrstUpwdDnwdTrgtPosCalib_TrgtPosArray_write) -> KeSMSw4SAcsMd25HdrstUpwdDnwdTrgtPosCalib_TrgtPosArray_write/1
  Subsystem1/4(KeSMSw4SAcsMd26HdrstUpwdDnwdTrgtPosCalib_TrgtPosArray_write) -> KeSMSw4SAcsMd26HdrstUpwdDnwdTrgtPosCalib_TrgtPosArray_write/1
  Subsystem1/5(LyLR2LHdrstUpwdDnwdTrgtPosCalib_TrgtPosArray_write) -> LyLR2LHdrstUpwdDnwdTrgtPosCalib_TrgtPosArray_write/1
  Subsystem1/6(RecvLR2LHdrstUpwdDnwdTrgtPosCalib_TrgtPosArray_write) -> RecvLR2LHdrstUpwdDnwdTrgtPosCalib_TrgtPosArray_write/1
  Subsystem1/7(VIPLR2LHdrstUpwdDnwdTrgtPosCalib_TrgtPosArray_write) -> VIPLR2LHdrstUpwdDnwdTrgtPosCalib_TrgtPosArray_write/1
  IfVeSMSuHeightIndexLt_Val_read/1 -> Subsystem1/1(IfVeSMSuHeightIndexLt_Val_read)
  StNumFlg_Is4s_read/1 -> Subsystem1/2(StNumFlg_Is4s_read)
  StNumFlg_Is6s_read/1 -> Subsystem1/3(StNumFlg_Is6s_read)
  StNumFlg_Is6s7s_read/1 -> Subsystem1/4(StNumFlg_Is6s7s_read)
  StNumFlg_Is7s_read/1 -> Subsystem1/5(StNumFlg_Is7s_read)

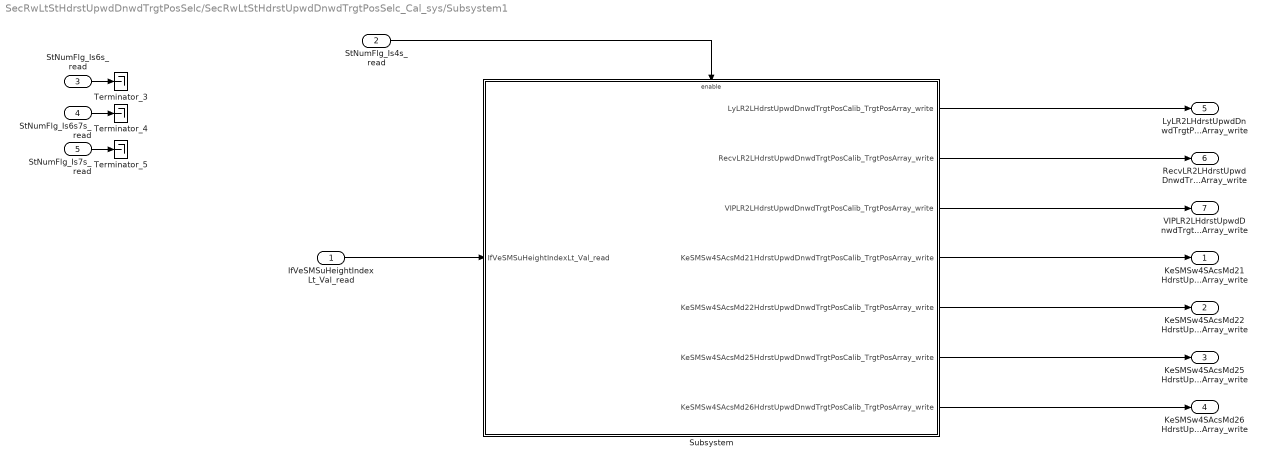
== system SecRwLtStHdrstUpwdDnwdTrgtPosSelc/SecRwLtStHdrstUpwdDnwdTrgtPosSelc_Cal_sys/Subsystem1 ==
  IfVeSMSuHeightIndexLt_Val_read : Inport
  StNumFlg_Is4s_read : Inport  Port=2
  StNumFlg_Is6s_read : Inport  Port=3
  StNumFlg_Is6s7s_read : Inport  Port=4
  StNumFlg_Is7s_read : Inport  Port=5
  Subsystem : Subsystem
  Terminator_3 : Terminator
  Terminator_4 : Terminator
  Terminator_5 : Terminator
  KeSMSw4SAcsMd21HdrstUpwdDnwdTrgtPosCalib_TrgtPosArray_write : Outport
      settings: EnsureOutportIsVirtual=on
  KeSMSw4SAcsMd22HdrstUpwdDnwdTrgtPosCalib_TrgtPosArray_write : Outport  Port=2
      settings: EnsureOutportIsVirtual=on
  KeSMSw4SAcsMd25HdrstUpwdDnwdTrgtPosCalib_TrgtPosArray_write : Outport  Port=3
      settings: EnsureOutportIsVirtual=on
  KeSMSw4SAcsMd26HdrstUpwdDnwdTrgtPosCalib_TrgtPosArray_write : Outport  Port=4
      settings: EnsureOutportIsVirtual=on
  LyLR2LHdrstUpwdDnwdTrgtPosCalib_TrgtPosArray_write : Outport  Port=5
      settings: EnsureOutportIsVirtual=on
  RecvLR2LHdrstUpwdDnwdTrgtPosCalib_TrgtPosArray_write : Outport  Port=6
      settings: EnsureOutportIsVirtual=on
  VIPLR2LHdrstUpwdDnwdTrgtPosCalib_TrgtPosArray_write : Outport  Port=7
      settings: EnsureOutportIsVirtual=on
  wires:
  IfVeSMSuHeightIndexLt_Val_read/1 -> Subsystem/1(IfVeSMSuHeightIndexLt_Val_read)
  StNumFlg_Is4s_read/1 -> Subsystem/Enable
  StNumFlg_Is6s_read/1 -> Terminator_3/1
  StNumFlg_Is6s7s_read/1 -> Terminator_4/1
  Subsystem/3(VIPLR2LHdrstUpwdDnwdTrgtPosCalib_TrgtPosArray_write) -> VIPLR2LHdrstUpwdDnwdTrgtPosCalib_TrgtPosArray_write/1
  Subsystem/2(RecvLR2LHdrstUpwdDnwdTrgtPosCalib_TrgtPosArray_write) -> RecvLR2LHdrstUpwdDnwdTrgtPosCalib_TrgtPosArray_write/1
  StNumFlg_Is7s_read/1 -> Terminator_5/1
  Subsystem/1(LyLR2LHdrstUpwdDnwdTrgtPosCalib_TrgtPosArray_write) -> LyLR2LHdrstUpwdDnwdTrgtPosCalib_TrgtPosArray_write/1
  Subsystem/6(KeSMSw4SAcsMd25HdrstUpwdDnwdTrgtPosCalib_TrgtPosArray_write) -> KeSMSw4SAcsMd25HdrstUpwdDnwdTrgtPosCalib_TrgtPosArray_write/1
  Subsystem/5(KeSMSw4SAcsMd22HdrstUpwdDnwdTrgtPosCalib_TrgtPosArray_write) -> KeSMSw4SAcsMd22HdrstUpwdDnwdTrgtPosCalib_TrgtPosArray_write/1
  Subsystem/7(KeSMSw4SAcsMd26HdrstUpwdDnwdTrgtPosCalib_TrgtPosArray_write) -> KeSMSw4SAcsMd26HdrstUpwdDnwdTrgtPosCalib_TrgtPosArray_write/1
  Subsystem/4(KeSMSw4SAcsMd21HdrstUpwdDnwdTrgtPosCalib_TrgtPosArray_write) -> KeSMSw4SAcsMd21HdrstUpwdDnwdTrgtPosCalib_TrgtPosArray_write/1

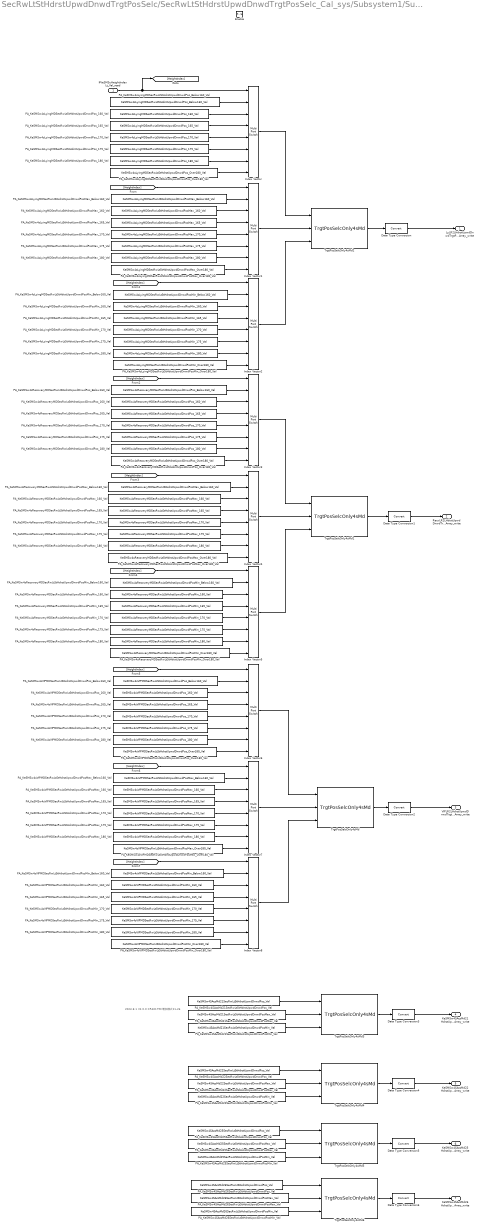
== system SecRwLtStHdrstUpwdDnwdTrgtPosSelc/SecRwLtStHdrstUpwdDnwdTrgtPosSelc_Cal_sys/Subsystem1/Subsystem ==
  note: 2023.8.1 V2.0.0 CR401790 增加模式21-26
  IfVeSMSuHeightIndexLt_Val_read : Inport
  Enable : EnablePort
  Data Type Conversion{,1..6} (7 alike) : DataTypeConversion
  Index Vector{,1..8} (9 alike) : MultiPortSwitch  DataPortOrder=Zero-based contiguous  Inputs=7  zeroidx=on
  PA_KeSMSw4SAcsMd21SecRwLtStHdrstUpwdDnwdPosMax_Val : Constant  Value=KeSMSw4SAcsMd21SecRwLtStHdrstUpwdDnwdPosMax_Val
  PA_KeSMSw4SAcsMd21SecRwLtStHdrstUpwdDnwdPosMin_Val : Constant  Value=KeSMSw4SAcsMd21SecRwLtStHdrstUpwdDnwdPosMin_Val
  PA_KeSMSw4SAcsMd21SecRwLtStHdrstUpwdDnwdPos_Val : Constant  Value=KeSMSw4SAcsMd21SecRwLtStHdrstUpwdDnwdPos_Val
  PA_KeSMSw4SAcsMd22SecRwLtStHdrstUpwdDnwdPosMax_Val : Constant  Value=KeSMSw4SAcsMd22SecRwLtStHdrstUpwdDnwdPosMax_Val
  PA_KeSMSw4SAcsMd22SecRwLtStHdrstUpwdDnwdPosMin_Val : Constant  Value=KeSMSw4SAcsMd22SecRwLtStHdrstUpwdDnwdPosMin_Val
  PA_KeSMSw4SAcsMd22SecRwLtStHdrstUpwdDnwdPos_Val : Constant  Value=KeSMSw4SAcsMd22SecRwLtStHdrstUpwdDnwdPos_Val
  PA_KeSMSw4SAcsMd25SecRwLtStHdrstUpwdDnwdPosMax_Val : Constant  Value=KeSMSw4SAcsMd25SecRwLtStHdrstUpwdDnwdPosMax_Val
  PA_KeSMSw4SAcsMd25SecRwLtStHdrstUpwdDnwdPosMin_Val : Constant  Value=KeSMSw4SAcsMd25SecRwLtStHdrstUpwdDnwdPosMin_Val
  PA_KeSMSw4SAcsMd25SecRwLtStHdrstUpwdDnwdPos_Val : Constant  Value=KeSMSw4SAcsMd25SecRwLtStHdrstUpwdDnwdPos_Val
  PA_KeSMSw4SAcsMd26SecRwLtStHdrstUpwdDnwdPosMax_Val : Constant  Value=KeSMSw4SAcsMd26SecRwLtStHdrstUpwdDnwdPosMax_Val
  PA_KeSMSw4SAcsMd26SecRwLtStHdrstUpwdDnwdPosMin_Val : Constant  Value=KeSMSw4SAcsMd26SecRwLtStHdrstUpwdDnwdPosMin_Val
  PA_KeSMSw4SAcsMd26SecRwLtStHdrstUpwdDnwdPos_Val : Constant  Value=KeSMSw4SAcsMd26SecRwLtStHdrstUpwdDnwdPos_Val
  PA_KeSMSw4sLyingMDSecRwLtStHdrstUpwdDnwdPosMax_160_Val : Constant  Value=KeSMSw4sLyingMDSecRwLtStHdrstUpwdDnwdPosMax_160_Val
  PA_KeSMSw4sLyingMDSecRwLtStHdrstUpwdDnwdPosMax_165_Val : Constant  Value=KeSMSw4sLyingMDSecRwLtStHdrstUpwdDnwdPosMax_165_Val
  PA_KeSMSw4sLyingMDSecRwLtStHdrstUpwdDnwdPosMax_170_Val : Constant  Value=KeSMSw4sLyingMDSecRwLtStHdrstUpwdDnwdPosMax_170_Val
  PA_KeSMSw4sLyingMDSecRwLtStHdrstUpwdDnwdPosMax_175_Val : Constant  Value=KeSMSw4sLyingMDSecRwLtStHdrstUpwdDnwdPosMax_175_Val
  PA_KeSMSw4sLyingMDSecRwLtStHdrstUpwdDnwdPosMax_180_Val : Constant  Value=KeSMSw4sLyingMDSecRwLtStHdrstUpwdDnwdPosMax_180_Val
  PA_KeSMSw4sLyingMDSecRwLtStHdrstUpwdDnwdPosMax_Below160_Val : Constant  Value=KeSMSw4sLyingMDSecRwLtStHdrstUpwdDnwdPosMax_Below160_Val
  PA_KeSMSw4sLyingMDSecRwLtStHdrstUpwdDnwdPosMax_Over180_Val : Constant  Value=KeSMSw4sLyingMDSecRwLtStHdrstUpwdDnwdPosMax_Over180_Val
  PA_KeSMSw4sLyingMDSecRwLtStHdrstUpwdDnwdPosMin_160_Val : Constant  Value=KeSMSw4sLyingMDSecRwLtStHdrstUpwdDnwdPosMin_160_Val
  PA_KeSMSw4sLyingMDSecRwLtStHdrstUpwdDnwdPosMin_165_Val : Constant  Value=KeSMSw4sLyingMDSecRwLtStHdrstUpwdDnwdPosMin_165_Val
  PA_KeSMSw4sLyingMDSecRwLtStHdrstUpwdDnwdPosMin_170_Val : Constant  Value=KeSMSw4sLyingMDSecRwLtStHdrstUpwdDnwdPosMin_170_Val
  PA_KeSMSw4sLyingMDSecRwLtStHdrstUpwdDnwdPosMin_175_Val : Constant  Value=KeSMSw4sLyingMDSecRwLtStHdrstUpwdDnwdPosMin_175_Val
  PA_KeSMSw4sLyingMDSecRwLtStHdrstUpwdDnwdPosMin_180_Val : Constant  Value=KeSMSw4sLyingMDSecRwLtStHdrstUpwdDnwdPosMin_180_Val
  PA_KeSMSw4sLyingMDSecRwLtStHdrstUpwdDnwdPosMin_Below160_Val : Constant  Value=KeSMSw4sLyingMDSecRwLtStHdrstUpwdDnwdPosMin_Below160_Val
  PA_KeSMSw4sLyingMDSecRwLtStHdrstUpwdDnwdPosMin_Over180_Val : Constant  Value=KeSMSw4sLyingMDSecRwLtStHdrstUpwdDnwdPosMin_Over180_Val
  PA_KeSMSw4sLyingMDSecRwLtStHdrstUpwdDnwdPos_160_Val : Constant  Value=KeSMSw4sLyingMDSecRwLtStHdrstUpwdDnwdPos_160_Val
  PA_KeSMSw4sLyingMDSecRwLtStHdrstUpwdDnwdPos_165_Val : Constant  Value=KeSMSw4sLyingMDSecRwLtStHdrstUpwdDnwdPos_165_Val
  PA_KeSMSw4sLyingMDSecRwLtStHdrstUpwdDnwdPos_170_Val : Constant  Value=KeSMSw4sLyingMDSecRwLtStHdrstUpwdDnwdPos_170_Val
  PA_KeSMSw4sLyingMDSecRwLtStHdrstUpwdDnwdPos_175_Val : Constant  Value=KeSMSw4sLyingMDSecRwLtStHdrstUpwdDnwdPos_175_Val
  PA_KeSMSw4sLyingMDSecRwLtStHdrstUpwdDnwdPos_180_Val : Constant  Value=KeSMSw4sLyingMDSecRwLtStHdrstUpwdDnwdPos_180_Val
  PA_KeSMSw4sLyingMDSecRwLtStHdrstUpwdDnwdPos_Below160_Val : Constant  Value=KeSMSw4sLyingMDSecRwLtStHdrstUpwdDnwdPos_Below160_Val
  PA_KeSMSw4sLyingMDSecRwLtStHdrstUpwdDnwdPos_Over180_Val : Constant  Value=KeSMSw4sLyingMDSecRwLtStHdrstUpwdDnwdPos_Over180_Val
  PA_KeSMSw4sRecoveryMDSecRwLtStHdrstUpwdDnwdPosMax_160_Val : Constant  Value=KeSMSw4sRecoveryMDSecRwLtStHdrstUpwdDnwdPosMax_160_Val
  PA_KeSMSw4sRecoveryMDSecRwLtStHdrstUpwdDnwdPosMax_165_Val : Constant  Value=KeSMSw4sRecoveryMDSecRwLtStHdrstUpwdDnwdPosMax_165_Val
  PA_KeSMSw4sRecoveryMDSecRwLtStHdrstUpwdDnwdPosMax_170_Val : Constant  Value=KeSMSw4sRecoveryMDSecRwLtStHdrstUpwdDnwdPosMax_170_Val
  PA_KeSMSw4sRecoveryMDSecRwLtStHdrstUpwdDnwdPosMax_175_Val : Constant  Value=KeSMSw4sRecoveryMDSecRwLtStHdrstUpwdDnwdPosMax_175_Val
  PA_KeSMSw4sRecoveryMDSecRwLtStHdrstUpwdDnwdPosMax_180_Val : Constant  Value=KeSMSw4sRecoveryMDSecRwLtStHdrstUpwdDnwdPosMax_180_Val
  PA_KeSMSw4sRecoveryMDSecRwLtStHdrstUpwdDnwdPosMax_Below160_Val : Constant  Value=KeSMSw4sRecoveryMDSecRwLtStHdrstUpwdDnwdPosMax_Below160_Val
  PA_KeSMSw4sRecoveryMDSecRwLtStHdrstUpwdDnwdPosMax_Over180_Val : Constant  Value=KeSMSw4sRecoveryMDSecRwLtStHdrstUpwdDnwdPosMax_Over180_Val
  PA_KeSMSw4sRecoveryMDSecRwLtStHdrstUpwdDnwdPosMin_160_Val : Constant  Value=KeSMSw4sRecoveryMDSecRwLtStHdrstUpwdDnwdPosMin_160_Val
  PA_KeSMSw4sRecoveryMDSecRwLtStHdrstUpwdDnwdPosMin_165_Val : Constant  Value=KeSMSw4sRecoveryMDSecRwLtStHdrstUpwdDnwdPosMin_165_Val
  PA_KeSMSw4sRecoveryMDSecRwLtStHdrstUpwdDnwdPosMin_170_Val : Constant  Value=KeSMSw4sRecoveryMDSecRwLtStHdrstUpwdDnwdPosMin_170_Val
  PA_KeSMSw4sRecoveryMDSecRwLtStHdrstUpwdDnwdPosMin_175_Val : Constant  Value=KeSMSw4sRecoveryMDSecRwLtStHdrstUpwdDnwdPosMin_175_Val
  PA_KeSMSw4sRecoveryMDSecRwLtStHdrstUpwdDnwdPosMin_180_Val : Constant  Value=KeSMSw4sRecoveryMDSecRwLtStHdrstUpwdDnwdPosMin_180_Val
  PA_KeSMSw4sRecoveryMDSecRwLtStHdrstUpwdDnwdPosMin_Below160_Val : Constant  Value=KeSMSw4sRecoveryMDSecRwLtStHdrstUpwdDnwdPosMin_Below160_Val
  PA_KeSMSw4sRecoveryMDSecRwLtStHdrstUpwdDnwdPosMin_Over180_Val : Constant  Value=KeSMSw4sRecoveryMDSecRwLtStHdrstUpwdDnwdPosMin_Over180_Val
  PA_KeSMSw4sRecoveryMDSecRwLtStHdrstUpwdDnwdPos_160_Val : Constant  Value=KeSMSw4sRecoveryMDSecRwLtStHdrstUpwdDnwdPos_160_Val
  PA_KeSMSw4sRecoveryMDSecRwLtStHdrstUpwdDnwdPos_165_Val : Constant  Value=KeSMSw4sRecoveryMDSecRwLtStHdrstUpwdDnwdPos_165_Val
  PA_KeSMSw4sRecoveryMDSecRwLtStHdrstUpwdDnwdPos_170_Val : Constant  Value=KeSMSw4sRecoveryMDSecRwLtStHdrstUpwdDnwdPos_170_Val
  PA_KeSMSw4sRecoveryMDSecRwLtStHdrstUpwdDnwdPos_175_Val : Constant  Value=KeSMSw4sRecoveryMDSecRwLtStHdrstUpwdDnwdPos_175_Val
  PA_KeSMSw4sRecoveryMDSecRwLtStHdrstUpwdDnwdPos_180_Val : Constant  Value=KeSMSw4sRecoveryMDSecRwLtStHdrstUpwdDnwdPos_180_Val
  PA_KeSMSw4sRecoveryMDSecRwLtStHdrstUpwdDnwdPos_Below160_Val : Constant  Value=KeSMSw4sRecoveryMDSecRwLtStHdrstUpwdDnwdPos_Below160_Val
  PA_KeSMSw4sRecoveryMDSecRwLtStHdrstUpwdDnwdPos_Over180_Val : Constant  Value=KeSMSw4sRecoveryMDSecRwLtStHdrstUpwdDnwdPos_Over180_Val
  PA_KeSMSw4sVIPMDSecRwLtStHdrstUpwdDnwdPosMax_160_Val : Constant  Value=KeSMSw4sVIPMDSecRwLtStHdrstUpwdDnwdPosMax_160_Val
  PA_KeSMSw4sVIPMDSecRwLtStHdrstUpwdDnwdPosMax_165_Val : Constant  Value=KeSMSw4sVIPMDSecRwLtStHdrstUpwdDnwdPosMax_165_Val
  PA_KeSMSw4sVIPMDSecRwLtStHdrstUpwdDnwdPosMax_170_Val : Constant  Value=KeSMSw4sVIPMDSecRwLtStHdrstUpwdDnwdPosMax_170_Val
  PA_KeSMSw4sVIPMDSecRwLtStHdrstUpwdDnwdPosMax_175_Val : Constant  Value=KeSMSw4sVIPMDSecRwLtStHdrstUpwdDnwdPosMax_175_Val
  PA_KeSMSw4sVIPMDSecRwLtStHdrstUpwdDnwdPosMax_180_Val : Constant  Value=KeSMSw4sVIPMDSecRwLtStHdrstUpwdDnwdPosMax_180_Val
  PA_KeSMSw4sVIPMDSecRwLtStHdrstUpwdDnwdPosMax_Below160_Val : Constant  Value=KeSMSw4sVIPMDSecRwLtStHdrstUpwdDnwdPosMax_Below160_Val
  PA_KeSMSw4sVIPMDSecRwLtStHdrstUpwdDnwdPosMax_Over180_Val : Constant  Value=KeSMSw4sVIPMDSecRwLtStHdrstUpwdDnwdPosMax_Over180_Val
  PA_KeSMSw4sVIPMDSecRwLtStHdrstUpwdDnwdPosMin_160_Val : Constant  Value=KeSMSw4sVIPMDSecRwLtStHdrstUpwdDnwdPosMin_160_Val
  PA_KeSMSw4sVIPMDSecRwLtStHdrstUpwdDnwdPosMin_165_Val : Constant  Value=KeSMSw4sVIPMDSecRwLtStHdrstUpwdDnwdPosMin_165_Val
  PA_KeSMSw4sVIPMDSecRwLtStHdrstUpwdDnwdPosMin_170_Val : Constant  Value=KeSMSw4sVIPMDSecRwLtStHdrstUpwdDnwdPosMin_170_Val
  PA_KeSMSw4sVIPMDSecRwLtStHdrstUpwdDnwdPosMin_175_Val : Constant  Value=KeSMSw4sVIPMDSecRwLtStHdrstUpwdDnwdPosMin_175_Val
  PA_KeSMSw4sVIPMDSecRwLtStHdrstUpwdDnwdPosMin_180_Val : Constant  Value=KeSMSw4sVIPMDSecRwLtStHdrstUpwdDnwdPosMin_180_Val
  PA_KeSMSw4sVIPMDSecRwLtStHdrstUpwdDnwdPosMin_Below160_Val : Constant  Value=KeSMSw4sVIPMDSecRwLtStHdrstUpwdDnwdPosMin_Below160_Val
  PA_KeSMSw4sVIPMDSecRwLtStHdrstUpwdDnwdPosMin_Over180_Val : Constant  Value=KeSMSw4sVIPMDSecRwLtStHdrstUpwdDnwdPosMin_Over180_Val
  PA_KeSMSw4sVIPMDSecRwLtStHdrstUpwdDnwdPos_160_Val : Constant  Value=KeSMSw4sVIPMDSecRwLtStHdrstUpwdDnwdPos_160_Val
  PA_KeSMSw4sVIPMDSecRwLtStHdrstUpwdDnwdPos_165_Val : Constant  Value=KeSMSw4sVIPMDSecRwLtStHdrstUpwdDnwdPos_165_Val
  PA_KeSMSw4sVIPMDSecRwLtStHdrstUpwdDnwdPos_170_Val : Constant  Value=KeSMSw4sVIPMDSecRwLtStHdrstUpwdDnwdPos_170_Val
  PA_KeSMSw4sVIPMDSecRwLtStHdrstUpwdDnwdPos_175_Val : Constant  Value=KeSMSw4sVIPMDSecRwLtStHdrstUpwdDnwdPos_175_Val
  PA_KeSMSw4sVIPMDSecRwLtStHdrstUpwdDnwdPos_180_Val : Constant  Value=KeSMSw4sVIPMDSecRwLtStHdrstUpwdDnwdPos_180_Val
  PA_KeSMSw4sVIPMDSecRwLtStHdrstUpwdDnwdPos_Below160_Val : Constant  Value=KeSMSw4sVIPMDSecRwLtStHdrstUpwdDnwdPos_Below160_Val
  PA_KeSMSw4sVIPMDSecRwLtStHdrstUpwdDnwdPos_Over180_Val : Constant  Value=KeSMSw4sVIPMDSecRwLtStHdrstUpwdDnwdPos_Over180_Val
  TrgtPosSelcOnly4sMd{,1..6} (7 alike) : TrgtPosSelcLib/TrgtPosSelcOnly4sMd  SystemSampleTime=-1
  LyLR2LHdrstUpwdDnwdTrgtPosCalib_TrgtPosArray_write : Outport
  RecvLR2LHdrstUpwdDnwdTrgtPosCalib_TrgtPosArray_write : Outport  Port=2
  VIPLR2LHdrstUpwdDnwdTrgtPosCalib_TrgtPosArray_write : Outport  Port=3
  KeSMSw4SAcsMd21HdrstUpwdDnwdTrgtPosCalib_TrgtPosArray_write : Outport  Port=4  InitialOutput=0
  KeSMSw4SAcsMd22HdrstUpwdDnwdTrgtPosCalib_TrgtPosArray_write : Outport  Port=5  InitialOutput=0
  KeSMSw4SAcsMd25HdrstUpwdDnwdTrgtPosCalib_TrgtPosArray_write : Outport  Port=6
  KeSMSw4SAcsMd26HdrstUpwdDnwdTrgtPosCalib_TrgtPosArray_write : Outport  Port=7
  wires:
  PA_KeSMSw4sLyingMDSecRwLtStHdrstUpwdDnwdPos_Below160_Val/1 -> Index Vector/2
  PA_KeSMSw4sLyingMDSecRwLtStHdrstUpwdDnwdPos_165_Val/1 -> Index Vector/4
  PA_KeSMSw4sVIPMDSecRwLtStHdrstUpwdDnwdPosMin_175_Val/1 -> Index Vector8/6
  PA_KeSMSw4sLyingMDSecRwLtStHdrstUpwdDnwdPosMin_Over180_Val/1 -> Index Vector2/8
  PA_KeSMSw4sRecoveryMDSecRwLtStHdrstUpwdDnwdPosMin_165_Val/1 -> Index Vector5/4
  [HeightIndex] -> Index Vector3/1
  Index Vector4/1 -> TrgtPosSelcOnly4sMd1/2
  Index Vector2/1 -> TrgtPosSelcOnly4sMd2/3
  PA_KeSMSw4sLyingMDSecRwLtStHdrstUpwdDnwdPos_Over180_Val/1 -> Index Vector/8
  [HeightIndex] -> Index Vector8/1
  Index Vector5/1 -> TrgtPosSelcOnly4sMd1/3
  PA_KeSMSw4sVIPMDSecRwLtStHdrstUpwdDnwdPosMax_Below160_Val/1 -> Index Vector7/2
  PA_KeSMSw4sVIPMDSecRwLtStHdrstUpwdDnwdPosMin_180_Val/1 -> Index Vector8/7
  PA_KeSMSw4sLyingMDSecRwLtStHdrstUpwdDnwdPos_175_Val/1 -> Index Vector/6
  PA_KeSMSw4sVIPMDSecRwLtStHdrstUpwdDnwdPosMax_160_Val/1 -> Index Vector7/3
  [HeightIndex] -> Index Vector2/1
  PA_KeSMSw4sVIPMDSecRwLtStHdrstUpwdDnwdPos_Below160_Val/1 -> Index Vector6/2
  [HeightIndex] -> Index Vector5/1
  PA_KeSMSw4sLyingMDSecRwLtStHdrstUpwdDnwdPos_160_Val/1 -> Index Vector/3
  TrgtPosSelcOnly4sMd1/1 -> Data Type Conversion1/1
  TrgtPosSelcOnly4sMd/1 -> Data Type Conversion2/1
  PA_KeSMSw4sVIPMDSecRwLtStHdrstUpwdDnwdPosMin_165_Val/1 -> Index Vector8/4
  PA_KeSMSw4sLyingMDSecRwLtStHdrstUpwdDnwdPosMax_Over180_Val/1 -> Index Vector1/8
  [HeightIndex] -> Index Vector1/1
  PA_KeSMSw4sRecoveryMDSecRwLtStHdrstUpwdDnwdPosMin_Over180_Val/1 -> Index Vector5/8
  IfVeSMSuHeightIndexLt_Val_read/1 -> [HeightIndex], Index Vector/1
  PA_KeSMSw4sRecoveryMDSecRwLtStHdrstUpwdDnwdPosMax_Below160_Val/1 -> Index Vector4/2
  PA_KeSMSw4sRecoveryMDSecRwLtStHdrstUpwdDnwdPos_175_Val/1 -> Index Vector3/6
  PA_KeSMSw4sLyingMDSecRwLtStHdrstUpwdDnwdPosMax_Below160_Val/1 -> Index Vector1/2
  PA_KeSMSw4sVIPMDSecRwLtStHdrstUpwdDnwdPos_175_Val/1 -> Index Vector6/6
  [HeightIndex] -> Index Vector6/1
  PA_KeSMSw4sRecoveryMDSecRwLtStHdrstUpwdDnwdPosMax_Over180_Val/1 -> Index Vector4/8
  PA_KeSMSw4sRecoveryMDSecRwLtStHdrstUpwdDnwdPosMin_175_Val/1 -> Index Vector5/6
  PA_KeSMSw4sRecoveryMDSecRwLtStHdrstUpwdDnwdPos_Below160_Val/1 -> Index Vector3/2
  PA_KeSMSw4sRecoveryMDSecRwLtStHdrstUpwdDnwdPos_180_Val/1 -> Index Vector3/7
  PA_KeSMSw4sRecoveryMDSecRwLtStHdrstUpwdDnwdPos_160_Val/1 -> Index Vector3/3
  PA_KeSMSw4sLyingMDSecRwLtStHdrstUpwdDnwdPosMax_165_Val/1 -> Index Vector1/4
  PA_KeSMSw4sVIPMDSecRwLtStHdrstUpwdDnwdPos_170_Val/1 -> Index Vector6/5
  PA_KeSMSw4sLyingMDSecRwLtStHdrstUpwdDnwdPosMax_160_Val/1 -> Index Vector1/3
  PA_KeSMSw4sRecoveryMDSecRwLtStHdrstUpwdDnwdPosMin_170_Val/1 -> Index Vector5/5
  PA_KeSMSw4sRecoveryMDSecRwLtStHdrstUpwdDnwdPos_Over180_Val/1 -> Index Vector3/8
  PA_KeSMSw4sLyingMDSecRwLtStHdrstUpwdDnwdPos_170_Val/1 -> Index Vector/5
  PA_KeSMSw4sRecoveryMDSecRwLtStHdrstUpwdDnwdPos_170_Val/1 -> Index Vector3/5
  PA_KeSMSw4sLyingMDSecRwLtStHdrstUpwdDnwdPosMin_165_Val/1 -> Index Vector2/4
  PA_KeSMSw4sRecoveryMDSecRwLtStHdrstUpwdDnwdPos_165_Val/1 -> Index Vector3/4
  PA_KeSMSw4sRecoveryMDSecRwLtStHdrstUpwdDnwdPosMin_180_Val/1 -> Index Vector5/7
  PA_KeSMSw4sLyingMDSecRwLtStHdrstUpwdDnwdPosMin_175_Val/1 -> Index Vector2/6
  PA_KeSMSw4sRecoveryMDSecRwLtStHdrstUpwdDnwdPosMax_170_Val/1 -> Index Vector4/5
  PA_KeSMSw4sRecoveryMDSecRwLtStHdrstUpwdDnwdPosMax_175_Val/1 -> Index Vector4/6
  PA_KeSMSw4sRecoveryMDSecRwLtStHdrstUpwdDnwdPosMax_165_Val/1 -> Index Vector4/4
  PA_KeSMSw4sRecoveryMDSecRwLtStHdrstUpwdDnwdPosMin_Below160_Val/1 -> Index Vector5/2
  PA_KeSMSw4sRecoveryMDSecRwLtStHdrstUpwdDnwdPosMax_180_Val/1 -> Index Vector4/7
  PA_KeSMSw4sRecoveryMDSecRwLtStHdrstUpwdDnwdPosMax_160_Val/1 -> Index Vector4/3
  PA_KeSMSw4sVIPMDSecRwLtStHdrstUpwdDnwdPos_180_Val/1 -> Index Vector6/7
  [HeightIndex] -> Index Vector4/1
  PA_KeSMSw4sLyingMDSecRwLtStHdrstUpwdDnwdPosMax_180_Val/1 -> Index Vector1/7
  PA_KeSMSw4sVIPMDSecRwLtStHdrstUpwdDnwdPos_Over180_Val/1 -> Index Vector6/8
  PA_KeSMSw4sVIPMDSecRwLtStHdrstUpwdDnwdPosMin_Over180_Val/1 -> Index Vector8/8
  Index Vector/1 -> TrgtPosSelcOnly4sMd2/1
  PA_KeSMSw4sVIPMDSecRwLtStHdrstUpwdDnwdPosMin_Below160_Val/1 -> Index Vector8/2
  PA_KeSMSw4sVIPMDSecRwLtStHdrstUpwdDnwdPosMax_165_Val/1 -> Index Vector7/4
  PA_KeSMSw4sVIPMDSecRwLtStHdrstUpwdDnwdPos_160_Val/1 -> Index Vector6/3
  PA_KeSMSw4sRecoveryMDSecRwLtStHdrstUpwdDnwdPosMin_160_Val/1 -> Index Vector5/3
  PA_KeSMSw4sLyingMDSecRwLtStHdrstUpwdDnwdPosMin_180_Val/1 -> Index Vector2/7
  [HeightIndex] -> Index Vector7/1
  Index Vector3/1 -> TrgtPosSelcOnly4sMd1/1
  PA_KeSMSw4sVIPMDSecRwLtStHdrstUpwdDnwdPosMin_170_Val/1 -> Index Vector8/5
  Index Vector7/1 -> TrgtPosSelcOnly4sMd/2
  PA_KeSMSw4sVIPMDSecRwLtStHdrstUpwdDnwdPosMax_Over180_Val/1 -> Index Vector7/8
  PA_KeSMSw4sLyingMDSecRwLtStHdrstUpwdDnwdPos_180_Val/1 -> Index Vector/7
  Index Vector1/1 -> TrgtPosSelcOnly4sMd2/2
  PA_KeSMSw4sVIPMDSecRwLtStHdrstUpwdDnwdPos_165_Val/1 -> Index Vector6/4
  PA_KeSMSw4sLyingMDSecRwLtStHdrstUpwdDnwdPosMin_Below160_Val/1 -> Index Vector2/2
  PA_KeSMSw4sLyingMDSecRwLtStHdrstUpwdDnwdPosMin_170_Val/1 -> Index Vector2/5
  TrgtPosSelcOnly4sMd2/1 -> Data Type Conversion/1
  PA_KeSMSw4sLyingMDSecRwLtStHdrstUpwdDnwdPosMax_170_Val/1 -> Index Vector1/5
  PA_KeSMSw4sVIPMDSecRwLtStHdrstUpwdDnwdPosMax_175_Val/1 -> Index Vector7/6
  PA_KeSMSw4sVIPMDSecRwLtStHdrstUpwdDnwdPosMin_160_Val/1 -> Index Vector8/3
  PA_KeSMSw4sVIPMDSecRwLtStHdrstUpwdDnwdPosMax_170_Val/1 -> Index Vector7/5
  Index Vector6/1 -> TrgtPosSelcOnly4sMd/1
  Index Vector8/1 -> TrgtPosSelcOnly4sMd/3
  PA_KeSMSw4sVIPMDSecRwLtStHdrstUpwdDnwdPosMax_180_Val/1 -> Index Vector7/7
  PA_KeSMSw4sLyingMDSecRwLtStHdrstUpwdDnwdPosMax_175_Val/1 -> Index Vector1/6
  PA_KeSMSw4sLyingMDSecRwLtStHdrstUpwdDnwdPosMin_160_Val/1 -> Index Vector2/3
  Data Type Conversion/1 -> LyLR2LHdrstUpwdDnwdTrgtPosCalib_TrgtPosArray_write/1
  Data Type Conversion1/1 -> RecvLR2LHdrstUpwdDnwdTrgtPosCalib_TrgtPosArray_write/1
  Data Type Conversion2/1 -> VIPLR2LHdrstUpwdDnwdTrgtPosCalib_TrgtPosArray_write/1
  TrgtPosSelcOnly4sMd4/1 -> Data Type Conversion4/1
  TrgtPosSelcOnly4sMd3/1 -> Data Type Conversion3/1
  TrgtPosSelcOnly4sMd5/1 -> Data Type Conversion5/1
  TrgtPosSelcOnly4sMd6/1 -> Data Type Conversion6/1
  PA_KeSMSw4SAcsMd26SecRwLtStHdrstUpwdDnwdPosMax_Val/1 -> TrgtPosSelcOnly4sMd6/2
  PA_KeSMSw4SAcsMd26SecRwLtStHdrstUpwdDnwdPosMin_Val/1 -> TrgtPosSelcOnly4sMd6/3
  PA_KeSMSw4SAcsMd26SecRwLtStHdrstUpwdDnwdPos_Val/1 -> TrgtPosSelcOnly4sMd6/1
  PA_KeSMSw4SAcsMd25SecRwLtStHdrstUpwdDnwdPosMax_Val/1 -> TrgtPosSelcOnly4sMd5/2
  PA_KeSMSw4SAcsMd25SecRwLtStHdrstUpwdDnwdPosMin_Val/1 -> TrgtPosSelcOnly4sMd5/3
  PA_KeSMSw4SAcsMd25SecRwLtStHdrstUpwdDnwdPos_Val/1 -> TrgtPosSelcOnly4sMd5/1
  PA_KeSMSw4SAcsMd22SecRwLtStHdrstUpwdDnwdPosMax_Val/1 -> TrgtPosSelcOnly4sMd4/2
  PA_KeSMSw4SAcsMd22SecRwLtStHdrstUpwdDnwdPosMin_Val/1 -> TrgtPosSelcOnly4sMd4/3
  PA_KeSMSw4SAcsMd22SecRwLtStHdrstUpwdDnwdPos_Val/1 -> TrgtPosSelcOnly4sMd4/1
  PA_KeSMSw4SAcsMd21SecRwLtStHdrstUpwdDnwdPosMax_Val/1 -> TrgtPosSelcOnly4sMd3/2
  PA_KeSMSw4SAcsMd21SecRwLtStHdrstUpwdDnwdPosMin_Val/1 -> TrgtPosSelcOnly4sMd3/3
  PA_KeSMSw4SAcsMd21SecRwLtStHdrstUpwdDnwdPos_Val/1 -> TrgtPosSelcOnly4sMd3/1
  Data Type Conversion3/1 -> KeSMSw4SAcsMd21HdrstUpwdDnwdTrgtPosCalib_TrgtPosArray_write/1
  Data Type Conversion4/1 -> KeSMSw4SAcsMd22HdrstUpwdDnwdTrgtPosCalib_TrgtPosArray_write/1
  Data Type Conversion5/1 -> KeSMSw4SAcsMd25HdrstUpwdDnwdTrgtPosCalib_TrgtPosArray_write/1
  Data Type Conversion6/1 -> KeSMSw4SAcsMd26HdrstUpwdDnwdTrgtPosCalib_TrgtPosArray_write/1
